simulink library "Variable_Frequency_Starter"  (R2024a)
settings: Solver=VariableStepAuto  StartTime=0.0  StopTime=10.0  RelTol=1e-3
libraries: spsDiodeLib x6, spsIGBTDiodeLib x6, spsThreePhaseParallelRLCBranchLib x3, spsThreePhaseBreakerLib x2, simulink x1, spsTriangleGeneratorLib x1, spsSeriesRLCBranchLib x1
settings Model: Creator=gshma  LastModifiedBy=gshma

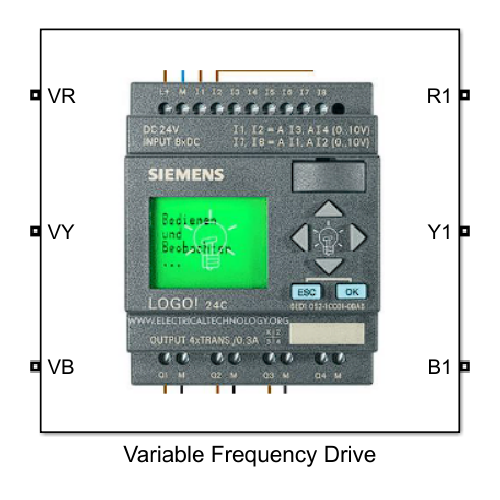
[thumbnail: Simulink's stored preview of the top-level diagram]
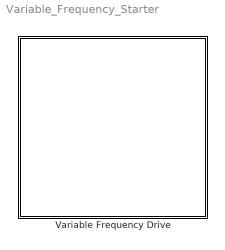
== system Variable_Frequency_Starter ==
  Variable Frequency Drive : Subsystem
      mask Display: image('control logic.png', [0,0,0,0,80,80]);

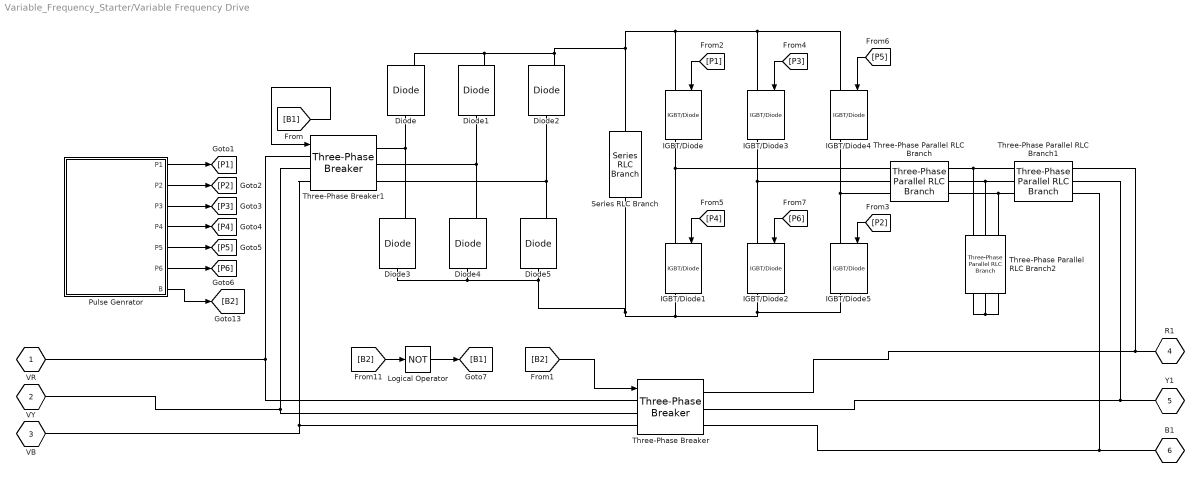
== system Variable_Frequency_Starter/Variable Frequency Drive ==
  Diode{,1..5} (6 alike) : spsDiodeLib/Diode  Ron=0.001  Lon=0  Vf=0.8  IC=0  UseSnubber=0  Rs=500  Cs=250e-9  Measurements=on
  IGBT/Diode{,1..5} (6 alike) : spsIGBTDiodeLib/IGBT//Diode  Ron=1e-3  Rs=1e5  Cs=inf  Measurements=on
  Logical Operator : Logic  Operator=NOT  AllPortsSameDT=off  OutDataTypeStr=boolean
  Pulse Genrator : Subsystem
  Series RLC Branch : spsSeriesRLCBranchLib/Series RLC Branch  LConnTagsString=__new0  RConnTagsString=__new0  BranchType=C  Resistance=1  Inductance=1e-3  SetiL0=off  InitialCurrent=0  Capacitance=7940*(10^-5)  Setx0=off  InitialVoltage=0  Measurements=None
  Three-Phase Parallel RLC Branch : spsThreePhaseParallelRLCBranchLib/Three-Phase Parallel RLC Branch  LConnTagsString=A|B|C  RConnTagsString=A|B|C  BranchType=L  Resistance=1  Inductance=2e-3  Capacitance=1e-6  Measurements=None
  Three-Phase Parallel RLC Branch1 : spsThreePhaseParallelRLCBranchLib/Three-Phase Parallel RLC Branch  LConnTagsString=A|B|C  RConnTagsString=A|B|C  BranchType=L  Resistance=1  Inductance=4e-3  Capacitance=1e-6  Measurements=None
  Three-Phase Parallel RLC Branch2 : spsThreePhaseParallelRLCBranchLib/Three-Phase Parallel RLC Branch  LConnTagsString=A|B|C  RConnTagsString=A|B|C  BranchType=C  Resistance=2  Inductance=5e-3  Capacitance=6e-6  Measurements=None
  Three-Phase Breaker : spsThreePhaseBreakerLib/Three-Phase Breaker  InitialState=open  SwitchA=on  SwitchB=on  SwitchC=on  SwitchTimes="[1/60  5/60]"  External=on  BreakerResistance=0.01  SnubberResistance=1e6  SnubberCapacitance=inf  Measurements=None
  Three-Phase Breaker1 : spsThreePhaseBreakerLib/Three-Phase Breaker  InitialState=closed  SwitchA=on  SwitchB=on  SwitchC=on  SwitchTimes="[1/60  5/60]"  External=on  BreakerResistance=0.01  SnubberResistance=1e6  SnubberCapacitance=inf  Measurements=None
  VR : PMIOPort  Tag=simrfV2util1/Connection Port  Side=Left
  VY : PMIOPort  Tag=simrfV2util1/Connection Port  Port=2  Side=Left
  VB : PMIOPort  Tag=simrfV2util1/Connection Port  Port=3  Side=Left
  R1 : PMIOPort  Tag=simrfV2util1/Connection Port  Port=4  Side=Right
  Y1 : PMIOPort  Tag=simrfV2util1/Connection Port  Port=5  Side=Right
  B1 : PMIOPort  Tag=simrfV2util1/Connection Port  Port=6  Side=Right
  wires:
  Pulse Genrator/1(P1) -> [P1]
  [P2] -> IGBT/Diode5/1
  [P6] -> IGBT/Diode2/1
  Pulse Genrator/4(P4) -> [P4]
  Pulse Genrator/5(P5) -> [P5]
  Logical Operator/1 -> [B1]
  [P4] -> IGBT/Diode1/1
  [B2] -> Three-Phase Breaker/1
  [P1] -> IGBT/Diode/1
  Pulse Genrator/6(P6) -> [P6]
  Pulse Genrator/3(P3) -> [P3]
  [P3] -> IGBT/Diode3/1
  [B1] -> Three-Phase Breaker1/1
  [P5] -> IGBT/Diode4/1
  Pulse Genrator/2(P2) -> [P2]
  [B2] -> Logical Operator/1
  Pulse Genrator/7(B) -> [B2]
  connections:
  Diode1/RConn1 -- Series RLC Branch/LConn1 -- IGBT/Diode/LConn1 -- IGBT/Diode4/LConn1 -- IGBT/Diode3/LConn1 -- Diode2/RConn1 -- Diode/RConn1
  Three-Phase Parallel RLC Branch1/LConn3 -- Three-Phase Parallel RLC Branch/RConn3 -- Three-Phase Parallel RLC Branch2/LConn3
  Three-Phase Parallel RLC Branch1/LConn1 -- Three-Phase Parallel RLC Branch/RConn1 -- Three-Phase Parallel RLC Branch2/LConn1
  Three-Phase Breaker/LConn3 -- Three-Phase Breaker1/LConn3 -- VB/RConn1
  IGBT/Diode2/RConn1 -- Series RLC Branch/RConn1 -- Diode4/LConn1 -- Diode3/LConn1 -- Diode5/LConn1 -- IGBT/Diode1/RConn1 -- IGBT/Diode5/RConn1
  Three-Phase Parallel RLC Branch1/LConn2 -- Three-Phase Parallel RLC Branch/RConn2 -- Three-Phase Parallel RLC Branch2/LConn2
  R1/RConn1 -- Three-Phase Breaker/RConn1 -- Three-Phase Parallel RLC Branch1/RConn1
  B1/RConn1 -- Three-Phase Breaker/RConn3 -- Three-Phase Parallel RLC Branch1/RConn3
  Three-Phase Breaker/LConn2 -- VY/RConn1 -- Three-Phase Breaker1/LConn2
  Three-Phase Parallel RLC Branch/LConn1 -- IGBT/Diode1/LConn1 -- IGBT/Diode/RConn1
  Three-Phase Breaker1/RConn3 -- Diode5/RConn1 -- Diode2/LConn1
  IGBT/Diode3/RConn1 -- IGBT/Diode2/LConn1 -- Three-Phase Parallel RLC Branch/LConn2
  Three-Phase Breaker1/LConn1 -- Three-Phase Breaker/LConn1 -- VR/RConn1
  Y1/RConn1 -- Three-Phase Breaker/RConn2 -- Three-Phase Parallel RLC Branch1/RConn2
  Three-Phase Parallel RLC Branch2/RConn2 -- Three-Phase Parallel RLC Branch2/RConn1 -- Three-Phase Parallel RLC Branch2/RConn3
  Three-Phase Breaker1/RConn2 -- Diode4/RConn1 -- Diode1/LConn1
  IGBT/Diode4/RConn1 -- IGBT/Diode5/LConn1 -- Three-Phase Parallel RLC Branch/LConn3
  Three-Phase Breaker1/RConn1 -- Diode3/RConn1 -- Diode/LConn1

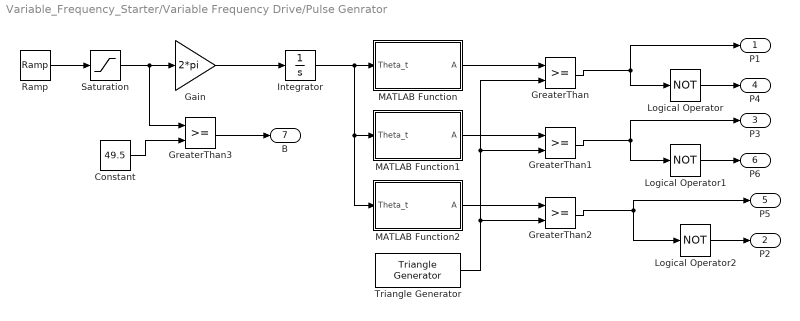
== system Variable_Frequency_Starter/Variable Frequency Drive/Pulse Genrator ==
  Constant : Constant  Value=49.5
  Gain : Gain  Gain=2*pi
  GreaterThan{,1..3} (4 alike) : RelationalOperator  OutDataTypeStr=boolean  RndMeth=Simplest  InputSameDT=off
  Integrator : Integrator
  Logical Operator : Logic  Operator=NOT  AllPortsSameDT=off  OutDataTypeStr=boolean
  Logical Operator1 : Logic  Operator=NOT  AllPortsSameDT=off  OutDataTypeStr=boolean
  Logical Operator2 : Logic  Operator=NOT  AllPortsSameDT=off  OutDataTypeStr=boolean
  MATLAB Function : MATLAB Function  TreatAsAtomicUnit=on
  MATLAB Function1 : MATLAB Function  TreatAsAtomicUnit=on
  MATLAB Function2 : MATLAB Function  TreatAsAtomicUnit=on
  Ramp : simulink/Sources/Ramp  slope=50/4  start=0  InitialOutput=0
  Saturation : Saturate  UpperLimit=50  LowerLimit=0
  Triangle Generator : spsTriangleGeneratorLib/Triangle Generator  Freq=20e3  Phase=90  Ts=0
  P1 : Outport
  P2 : Outport  Port=2
  P3 : Outport  Port=3
  P4 : Outport  Port=4
  P5 : Outport  Port=5
  P6 : Outport  Port=6
  B : Outport  Port=7
  wires:
  Logical Operator1/1 -> P6/1
  Logical Operator2/1 -> P2/1
  Logical Operator/1 -> P4/1
  GreaterThan/1 -> P1/1, Logical Operator/1
  MATLAB Function1/1(A) -> GreaterThan1/1
  Gain/1 -> Integrator/1
  MATLAB Function2/1(A) -> GreaterThan2/1
  GreaterThan2/1 -> P5/1, Logical Operator2/1
  Integrator/1 -> MATLAB Function2/1(Theta_t), MATLAB Function1/1(Theta_t), MATLAB Function/1(Theta_t)
  Saturation/1 -> GreaterThan3/1, Gain/1
  Ramp/1 -> Saturation/1
  GreaterThan1/1 -> Logical Operator1/1, P3/1
  MATLAB Function/1(A) -> GreaterThan/1
  Triangle Generator/1 -> GreaterThan1/2, GreaterThan/2, GreaterThan2/2
  Constant/1 -> GreaterThan3/2
  GreaterThan3/1 -> B/1

== matlab function Variable_Frequency_Starter/Variable Frequency Drive/Pulse Genrator/MATLAB Function ==
  data: Theta_t input; A output
function A = SineA(Theta_t)
A = sin(Theta_t);
end

== matlab function Variable_Frequency_Starter/Variable Frequency Drive/Pulse Genrator/MATLAB Function2 ==
  data: Theta_t input; A output
function A = SineC(Theta_t)
A = sin(Theta_t-2*pi/3);
end

== matlab function Variable_Frequency_Starter/Variable Frequency Drive/Pulse Genrator/MATLAB Function1 ==
  data: Theta_t input; A output
function A = SineB(Theta_t)
A = sin(Theta_t+2*pi/3);
end
